simulink model "Catch_traffic_light_ver05_sushi_201222"  (R2019b)
settings: Solver=ode1  StartTime=0.0  StopTime=inf  FixedStep=0.001  RelTol=1e-3
PreLoadFcn:
  | vehicle = 'Car'; if ~length(which('cmself')), cmenv; end
  | Catch_traffic_light_ver02_sushi_201217_bus
InitFcn:
  | vehicle = 'Car'; if ~length(which('cmself')), cmenv; end
  | Catch_traffic_light_ver02_sushi_201217_bus
libraries: CarMaker4SL x45, simulink x3
Description:
  | CarMaker Plug-in Model Target
settings Model: Creator=ambl  LastModifiedBy=ambl
settings RTWCC: Description=CarMaker Plug-in Model Target  SystemTargetFile=CarMaker.tlc  TemplateMakefile=CarMaker_unix-linux64.tmf
settings CodeAppCC: MaxIdLength=127
settings STFCustomTargetCC: TargetLangStandard=C99 (ISO)  CombineOutputUpdateFcns=on  MultiInstanceERTCode=on  CodeInterfacePackaging=Reusable function  GenerateAllocFcn=on  SystemTargetFile=CarMaker.tlc
settings GRTTargetCC: ParMdlRefBuildCompliant=off  CompOptLevelCompliant=off  ConcurrentExecutionCompliant=off  MatFileLogging=off  MultiInstanceERTCode=on  CodeInterfacePackaging=Reusable function  CPPClassGenCompliant=off  GenerateAllocFcn=on  UseToolchainInfoCompliant=off

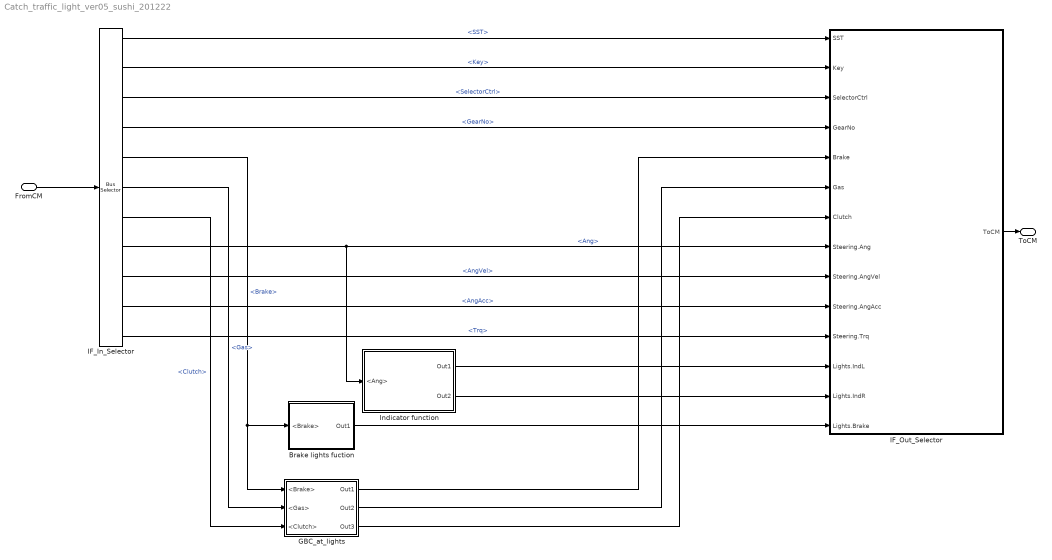
== system Catch_traffic_light_ver05_sushi_201222 ==
  FromCM : Inport  OutDataTypeStr=Bus: cmVehicleControlIn
  Brake lights fuction : Subsystem
  GBC_at_lights : Subsystem
  IF_In_Selector : BusSelector  OutputSignals=SST,Key,SelectorCtrl,GearNo,Brake,Gas,Clutch,Steering.Ang,Steering.AngVel,Steering.AngAcc,Steering.Trq
  IF_Out_Selector : Subsystem  mask(Signal Selection){}
      mask help: Signal Selection Block
      settings: OpenFcn=cmSignalSelect('SignalSelection_CB',gcb)
  Indicator function : Subsystem
  ToCM : Outport  OutDataTypeStr=Bus: cmVehicleControlOut
  wires:
  FromCM/1 -> IF_In_Selector/1
  IF_Out_Selector/1(ToCM) -> ToCM/1
  IF_In_Selector/1 -> IF_Out_Selector/1(SST)  "<SST>"
  IF_In_Selector/2 -> IF_Out_Selector/2(Key)  "<Key>"
  IF_In_Selector/3 -> IF_Out_Selector/3(SelectorCtrl)  "<SelectorCtrl>"
  IF_In_Selector/5 -> Brake lights fuction/1(<Brake>), GBC_at_lights/1(<Brake>)  "<Brake>"
  IF_In_Selector/8 -> IF_Out_Selector/8(Steering.Ang), Indicator function/1("<Ang> ")  "<Ang>"
  IF_In_Selector/9 -> IF_Out_Selector/9(Steering.AngVel)  "<AngVel>"
  IF_In_Selector/10 -> IF_Out_Selector/10(Steering.AngAcc)  "<AngAcc>"
  IF_In_Selector/11 -> IF_Out_Selector/11(Steering.Trq)  "<Trq>"
  Brake lights fuction/1(Out1) -> IF_Out_Selector/14(Lights.Brake)
  Indicator function/1(Out1) -> IF_Out_Selector/12(Lights.IndL)
  Indicator function/2(Out2) -> IF_Out_Selector/13(Lights.IndR)
  IF_In_Selector/6 -> GBC_at_lights/2(<Gas>)  "<Gas>"
  IF_In_Selector/7 -> GBC_at_lights/3(<Clutch>)  "<Clutch>"
  GBC_at_lights/3(Out3) -> IF_Out_Selector/7(Clutch)
  GBC_at_lights/2(Out2) -> IF_Out_Selector/6(Gas)
  GBC_at_lights/1(Out1) -> IF_Out_Selector/5(Brake)
  IF_In_Selector/4 -> IF_Out_Selector/4(GearNo)  "<GearNo>"

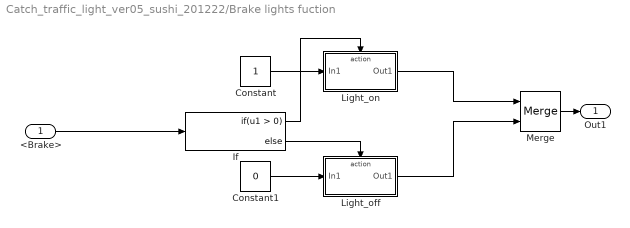
== system Catch_traffic_light_ver05_sushi_201222/Brake lights fuction ==
  <Brake> : Inport
  Constant : Constant
  Constant1 : Constant  Value=0
  If : If
  Light_off : Subsystem  TreatAsAtomicUnit=on
  Light_on : Subsystem  TreatAsAtomicUnit=on
  Merge : Merge
  Out1 : Outport
  wires:
  If/2 -> Light_off/Action
  Constant1/1 -> Light_off/1(In1)
  Merge/1 -> Out1/1
  Constant/1 -> Light_on/1(In1)
  <Brake>/1 -> If/1
  Light_on/1(Out1) -> Merge/1
  Light_off/1(Out1) -> Merge/2
  If/1 -> Light_on/Action

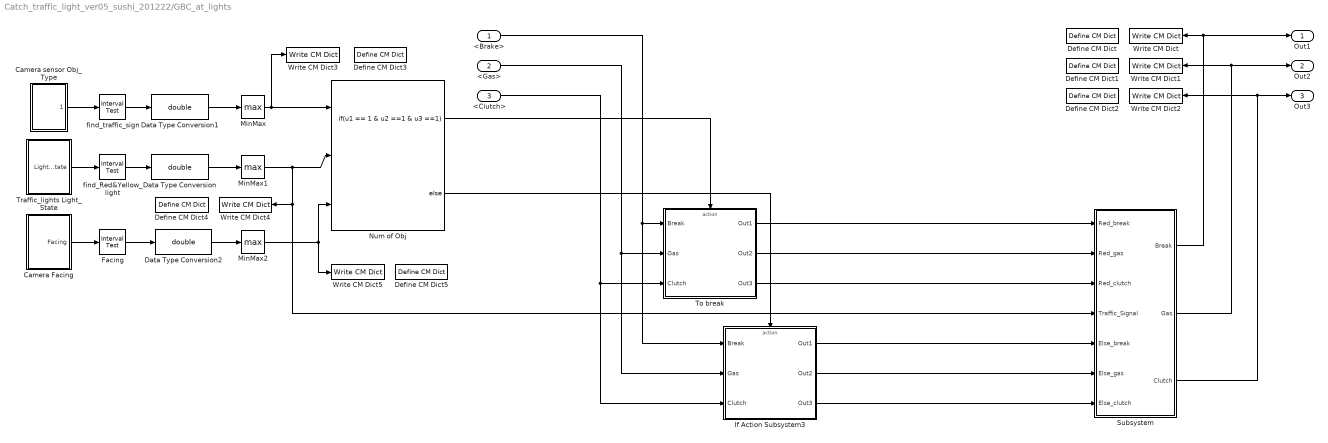
== system Catch_traffic_light_ver05_sushi_201222/GBC_at_lights ==
  <Brake> : Inport
  <Gas> : Inport  Port=2
  <Clutch> : Inport  Port=3
  Camera Facing : Subsystem
  Camera sensor Obj_Type : Subsystem
  Data Type Conversion : DataTypeConversion  OutDataTypeStr=double
  Data Type Conversion1 : DataTypeConversion  OutDataTypeStr=double
  Data Type Conversion2 : DataTypeConversion  OutDataTypeStr=double
  Define CM Dict : CarMaker4SL/Define CM Dict  xname=ctrl_break  xmono=off  xtype=Double4  xdvaplace=None  xnstates=0  xfirststate=0  xinitial=0
  Define CM Dict1 : CarMaker4SL/Define CM Dict  xname=ctrl_gas  xmono=off  xtype=Double4  xdvaplace=None  xnstates=0  xfirststate=0  xinitial=0
  Define CM Dict2 : CarMaker4SL/Define CM Dict  xname=ctrl_clutch  xmono=off  xtype=Double4  xdvaplace=None  xnstates=0  xfirststate=0  xinitial=0
  Define CM Dict3 : CarMaker4SL/Define CM Dict  xname=ctrl_obj_type  xmono=off  xtype=Double4  xdvaplace=None  xnstates=0  xfirststate=0  xinitial=0
  Define CM Dict4 : CarMaker4SL/Define CM Dict  xname=ctrl_light_state  xmono=off  xtype=Double4  xdvaplace=None  xnstates=0  xfirststate=0  xinitial=0
  Define CM Dict5 : CarMaker4SL/Define CM Dict  xname=ctrl_facing  xmono=off  xtype=Double4  xdvaplace=None  xnstates=0  xfirststate=0  xinitial=0
  Facing : simulink/Logic and Bit Operations/Interval Test  IntervalClosedRight=on  uplimit=1.5  IntervalClosedLeft=on  lowlimit=0.5  OutDataTypeStr=boolean
  If Action Subsystem3 : Subsystem  TreatAsAtomicUnit=on
  MinMax : MinMax  Function=max
  MinMax1 : MinMax  Function=max
  MinMax2 : MinMax  Function=max
  Num of Obj : If  NumInputs=3  IfExpression=u1 == 1 & u2 ==1 & u3 ==1
  Subsystem : Subsystem
  To break : Subsystem  TreatAsAtomicUnit=on
  Traffic_lights Light_State : Subsystem
  Write CM Dict : CarMaker4SL/Write CM Dict  xname=ctrl_break  xsync=off
  Write CM Dict1 : CarMaker4SL/Write CM Dict  xname=ctrl_gas  xsync=off
  Write CM Dict2 : CarMaker4SL/Write CM Dict  xname=ctrl_clutch  xsync=off
  Write CM Dict3 : CarMaker4SL/Write CM Dict  xname=ctrl_obj_type  xsync=off
  Write CM Dict4 : CarMaker4SL/Write CM Dict  xname=ctrl_light_state  xsync=off
  Write CM Dict5 : CarMaker4SL/Write CM Dict  xname=ctrl_facing  xsync=off
  find_Red&Yellow_light : simulink/Logic and Bit Operations/Interval Test  IntervalClosedRight=on  uplimit=3.5  IntervalClosedLeft=on  lowlimit=2.5  OutDataTypeStr=boolean
  find_traffic_sign : simulink/Logic and Bit Operations/Interval Test  IntervalClosedRight=on  uplimit=5.5  IntervalClosedLeft=on  lowlimit=4.5  OutDataTypeStr=boolean
  Out1 : Outport
  Out2 : Outport  Port=2
  Out3 : Outport  Port=3
  wires:
  Subsystem/2(Gas) -> Write CM Dict1/1, Out2/1
  Subsystem/1(Break) -> Write CM Dict/1, Out1/1
  Subsystem/3(Clutch) -> Write CM Dict2/1, Out3/1
  If Action Subsystem3/1(Out1) -> Subsystem/5(Else_break)
  If Action Subsystem3/2(Out2) -> Subsystem/6("Else_gas ")
  If Action Subsystem3/3(Out3) -> Subsystem/7("Else_clutch ")
  To break/1(Out1) -> Subsystem/1(Red_break)
  To break/2(Out2) -> Subsystem/2(Red_gas)
  To break/3(Out3) -> Subsystem/3(Red_clutch)
  Num of Obj/1 -> To break/Action
  Num of Obj/2 -> If Action Subsystem3/Action
  <Gas>/1 -> If Action Subsystem3/2(Gas), To break/2(Gas)
  <Brake>/1 -> If Action Subsystem3/1(Break), To break/1(Break)
  <Clutch>/1 -> If Action Subsystem3/3(Clutch), To break/3(Clutch)
  find_traffic_sign/1 -> Data Type Conversion1/1
  Camera sensor Obj_Type/1(Obj_Type) -> find_traffic_sign/1
  Traffic_lights Light_State/1(Light_State) -> find_Red&Yellow_light/1
  MinMax/1 -> Write CM Dict3/1, Num of Obj/1
  MinMax1/1 -> Subsystem/4(Traffic_Signal), Write CM Dict4/1, Num of Obj/2
  Data Type Conversion1/1 -> MinMax/1
  find_Red&Yellow_light/1 -> Data Type Conversion/1
  Data Type Conversion/1 -> MinMax1/1
  Camera Facing/1(Facing) -> Facing/1
  Facing/1 -> Data Type Conversion2/1
  Data Type Conversion2/1 -> MinMax2/1
  MinMax2/1 -> Write CM Dict5/1, Num of Obj/3

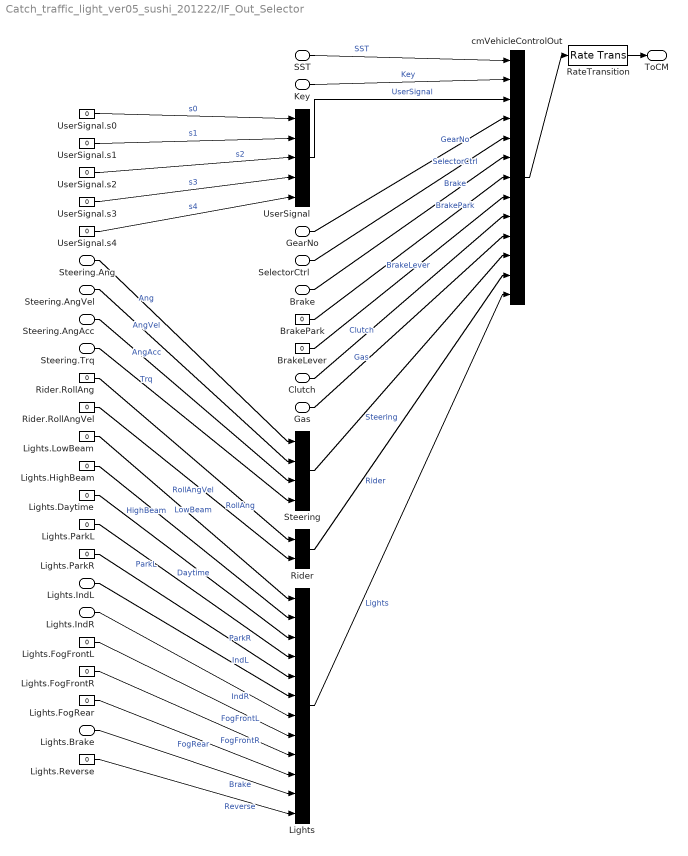
== system Catch_traffic_light_ver05_sushi_201222/IF_Out_Selector ==
  SST : Inport
  Key : Inport  Port=2
  SelectorCtrl : Inport  Port=3
  GearNo : Inport  Port=4
  Brake : Inport  Port=5
  Gas : Inport  Port=6
  Clutch : Inport  Port=7
  Steering.Ang : Inport  Port=8
  Steering.AngVel : Inport  Port=9
  Steering.AngAcc : Inport  Port=10
  Steering.Trq : Inport  Port=11
  Lights.IndL : Inport  Port=12
  Lights.IndR : Inport  Port=13
  Lights.Brake : Inport  Port=14
  BrakeLever : Constant  Value=0
  BrakePark : Constant  Value=0
  Lights : BusCreator  Inputs=12
  Lights.Daytime : Constant  Value=0
  Lights.FogFrontL : Constant  Value=0
  Lights.FogFrontR : Constant  Value=0
  Lights.FogRear : Constant  Value=0
  Lights.HighBeam : Constant  Value=0
  Lights.LowBeam : Constant  Value=0
  Lights.ParkL : Constant  Value=0
  Lights.ParkR : Constant  Value=0
  Lights.Reverse : Constant  Value=0
  RateTransition : RateTransition  OutPortSampleTime=str2num(get_param(bdroot,'FixedStep'))
  Rider : BusCreator  Inputs=2
  Rider.RollAng : Constant  Value=0
  Rider.RollAngVel : Constant  Value=0
  Steering : BusCreator  Inputs=4
  UserSignal : BusCreator  Inputs=5
  UserSignal.s{0..4} (5 alike) : Constant  Value=0
  cmVehicleControlOut : BusCreator  Inputs=13
  ToCM : Outport
  wires:
  RateTransition/1 -> ToCM/1
  cmVehicleControlOut/1 -> RateTransition/1
  UserSignal/1 -> cmVehicleControlOut/3  "UserSignal"
  UserSignal.s0/1 -> UserSignal/1  "s0"
  UserSignal.s1/1 -> UserSignal/2  "s1"
  UserSignal.s2/1 -> UserSignal/3  "s2"
  UserSignal.s3/1 -> UserSignal/4  "s3"
  UserSignal.s4/1 -> UserSignal/5  "s4"
  BrakePark/1 -> cmVehicleControlOut/7  "BrakePark"
  BrakeLever/1 -> cmVehicleControlOut/8  "BrakeLever"
  Steering/1 -> cmVehicleControlOut/11  "Steering"
  Rider/1 -> cmVehicleControlOut/12  "Rider"
  Rider.RollAng/1 -> Rider/1  "RollAng"
  Rider.RollAngVel/1 -> Rider/2  "RollAngVel"
  Lights/1 -> cmVehicleControlOut/13  "Lights"
  Lights.LowBeam/1 -> Lights/1  "LowBeam"
  Lights.HighBeam/1 -> Lights/2  "HighBeam"
  Lights.Daytime/1 -> Lights/3  "Daytime"
  Lights.ParkL/1 -> Lights/4  "ParkL"
  Lights.ParkR/1 -> Lights/5  "ParkR"
  Lights.FogFrontL/1 -> Lights/8  "FogFrontL"
  Lights.FogFrontR/1 -> Lights/9  "FogFrontR"
  Lights.FogRear/1 -> Lights/10  "FogRear"
  Lights.Reverse/1 -> Lights/12  "Reverse"
  SST/1 -> cmVehicleControlOut/1  "SST"
  Key/1 -> cmVehicleControlOut/2  "Key"
  GearNo/1 -> cmVehicleControlOut/4  "GearNo"
  SelectorCtrl/1 -> cmVehicleControlOut/5  "SelectorCtrl"
  Brake/1 -> cmVehicleControlOut/6  "Brake"
  Clutch/1 -> cmVehicleControlOut/9  "Clutch"
  Gas/1 -> cmVehicleControlOut/10  "Gas"
  Steering.Ang/1 -> Steering/1  "Ang"
  Steering.AngVel/1 -> Steering/2  "AngVel"
  Steering.AngAcc/1 -> Steering/3  "AngAcc"
  Steering.Trq/1 -> Steering/4  "Trq"
  Lights.IndL/1 -> Lights/6  "IndL"
  Lights.IndR/1 -> Lights/7  "IndR"
  Lights.Brake/1 -> Lights/11  "Brake"

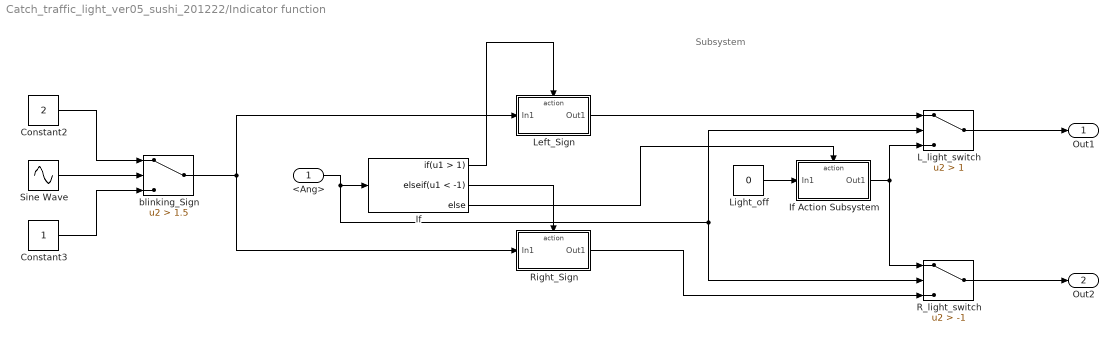
== system Catch_traffic_light_ver05_sushi_201222/Indicator function ==
  note: Subsystem
  "<Ang> " : Inport
  Constant2 : Constant  Value=2
  Constant3 : Constant
  If : If  IfExpression=u1 > 1  ElseIfExpressions=u1 < -1
  If Action Subsystem : Subsystem  TreatAsAtomicUnit=on
  L_light_switch : Switch  Criteria=u2 > Threshold  Threshold=1
  Left_Sign : Subsystem  TreatAsAtomicUnit=on
  Light_off : Constant  Value=0
  R_light_switch : Switch  Criteria=u2 > Threshold  Threshold=-1
  Right_Sign : Subsystem  TreatAsAtomicUnit=on
  Sine Wave : Sin  Amplitude=0.5  Bias=1.5  Frequency=4.71  SampleTime=0
  blinking_Sign : Switch  Criteria=u2 > Threshold  Threshold=1.5
  Out1 : Outport
  Out2 : Outport  Port=2
  wires:
  If/1 -> Left_Sign/Action
  Sine Wave/1 -> blinking_Sign/2
  Constant2/1 -> blinking_Sign/1
  Constant3/1 -> blinking_Sign/3
  blinking_Sign/1 -> Left_Sign/1(In1), Right_Sign/1(In1)
  If/2 -> Right_Sign/Action
  L_light_switch/1 -> Out1/1
  R_light_switch/1 -> Out2/1
  "<Ang> "/1 -> L_light_switch/2, R_light_switch/2, If/1
  Light_off/1 -> If Action Subsystem/1(In1)
  If Action Subsystem/1(Out1) -> R_light_switch/1, L_light_switch/3
  Right_Sign/1(Out1) -> R_light_switch/3
  Left_Sign/1(Out1) -> L_light_switch/1
  If/3 -> If Action Subsystem/Action

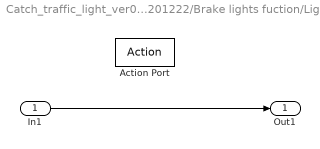
== system Catch_traffic_light_ver05_sushi_201222/Brake lights fuction/Light_off ==
  In1 : Inport
  Action Port : ActionPort  ActionPortLabel=else
  Out1 : Outport
  wires:
  In1/1 -> Out1/1

== system Catch_traffic_light_ver05_sushi_201222/Brake lights fuction/Light_on ==
  In1 : Inport
  Action Port : ActionPort  ActionPortLabel=if(u1 > 0)
  Out1 : Outport
  wires:
  In1/1 -> Out1/1

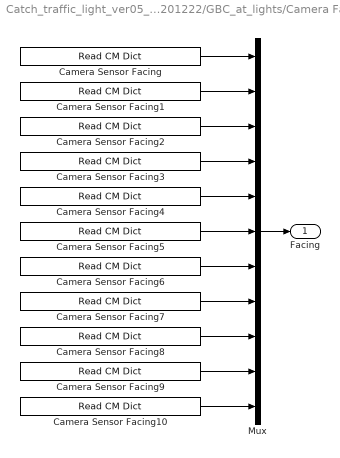
== system Catch_traffic_light_ver05_sushi_201222/GBC_at_lights/Camera Facing ==
  Camera Sensor Facing : CarMaker4SL/Read CM Dict  xname=Sensor.Camera.CA00.Obj.0.Facing  xsync=off
  Camera Sensor Facing1 : CarMaker4SL/Read CM Dict  xname=Sensor.Camera.CA00.Obj.1.Facing  xsync=off
  Camera Sensor Facing10 : CarMaker4SL/Read CM Dict  xname=Sensor.Camera.CA00.Obj.10.Facing  xsync=off
  Camera Sensor Facing2 : CarMaker4SL/Read CM Dict  xname=Sensor.Camera.CA00.Obj.2.Facing  xsync=off
  Camera Sensor Facing3 : CarMaker4SL/Read CM Dict  xname=Sensor.Camera.CA00.Obj.3.Facing  xsync=off
  Camera Sensor Facing4 : CarMaker4SL/Read CM Dict  xname=Sensor.Camera.CA00.Obj.4.Facing  xsync=off
  Camera Sensor Facing5 : CarMaker4SL/Read CM Dict  xname=Sensor.Camera.CA00.Obj.5.Facing  xsync=off
  Camera Sensor Facing6 : CarMaker4SL/Read CM Dict  xname=Sensor.Camera.CA00.Obj.6.Facing  xsync=off
  Camera Sensor Facing7 : CarMaker4SL/Read CM Dict  xname=Sensor.Camera.CA00.Obj.7.Facing  xsync=off
  Camera Sensor Facing8 : CarMaker4SL/Read CM Dict  xname=Sensor.Camera.CA00.Obj.8.Facing  xsync=off
  Camera Sensor Facing9 : CarMaker4SL/Read CM Dict  xname=Sensor.Camera.CA00.Obj.9.Facing  xsync=off
  Mux : Mux  Inputs=11
  Facing : Outport
  wires:
  Camera Sensor Facing/1 -> Mux/1
  Camera Sensor Facing1/1 -> Mux/2
  Camera Sensor Facing2/1 -> Mux/3
  Camera Sensor Facing3/1 -> Mux/4
  Camera Sensor Facing4/1 -> Mux/5
  Camera Sensor Facing5/1 -> Mux/6
  Camera Sensor Facing6/1 -> Mux/7
  Camera Sensor Facing7/1 -> Mux/8
  Camera Sensor Facing8/1 -> Mux/9
  Camera Sensor Facing9/1 -> Mux/10
  Camera Sensor Facing10/1 -> Mux/11
  Mux/1 -> Facing/1

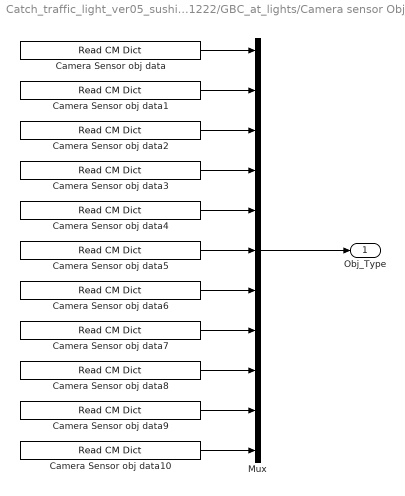
== system Catch_traffic_light_ver05_sushi_201222/GBC_at_lights/Camera sensor Obj_Type ==
  Camera Sensor obj data : CarMaker4SL/Read CM Dict  xname=Sensor.Camera.CA00.Obj.0.Type  xsync=off
  Camera Sensor obj data1 : CarMaker4SL/Read CM Dict  xname=Sensor.Camera.CA00.Obj.1.Type  xsync=off
  Camera Sensor obj data10 : CarMaker4SL/Read CM Dict  xname=Sensor.Camera.CA00.Obj.10.Type  xsync=off
  Camera Sensor obj data2 : CarMaker4SL/Read CM Dict  xname=Sensor.Camera.CA00.Obj.2.Type  xsync=off
  Camera Sensor obj data3 : CarMaker4SL/Read CM Dict  xname=Sensor.Camera.CA00.Obj.3.Type  xsync=off
  Camera Sensor obj data4 : CarMaker4SL/Read CM Dict  xname=Sensor.Camera.CA00.Obj.4.Type  xsync=off
  Camera Sensor obj data5 : CarMaker4SL/Read CM Dict  xname=Sensor.Camera.CA00.Obj.5.Type  xsync=off
  Camera Sensor obj data6 : CarMaker4SL/Read CM Dict  xname=Sensor.Camera.CA00.Obj.6.Type  xsync=off
  Camera Sensor obj data7 : CarMaker4SL/Read CM Dict  xname=Sensor.Camera.CA00.Obj.7.Type  xsync=off
  Camera Sensor obj data8 : CarMaker4SL/Read CM Dict  xname=Sensor.Camera.CA00.Obj.8.Type  xsync=off
  Camera Sensor obj data9 : CarMaker4SL/Read CM Dict  xname=Sensor.Camera.CA00.Obj.9.Type  xsync=off
  Mux : Mux  Inputs=11
  Obj_Type : Outport
  wires:
  Camera Sensor obj data6/1 -> Mux/7
  Camera Sensor obj data7/1 -> Mux/8
  Camera Sensor obj data3/1 -> Mux/4
  Camera Sensor obj data/1 -> Mux/1
  Camera Sensor obj data5/1 -> Mux/6
  Camera Sensor obj data2/1 -> Mux/3
  Camera Sensor obj data10/1 -> Mux/11
  Camera Sensor obj data1/1 -> Mux/2
  Camera Sensor obj data8/1 -> Mux/9
  Camera Sensor obj data4/1 -> Mux/5
  Camera Sensor obj data9/1 -> Mux/10
  Mux/1 -> Obj_Type/1

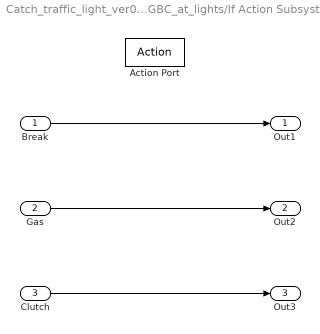
== system Catch_traffic_light_ver05_sushi_201222/GBC_at_lights/If Action Subsystem3 ==
  Break : Inport
  Gas : Inport  Port=2
  Clutch : Inport  Port=3
  Action Port : ActionPort  ActionPortLabel=else
  Out1 : Outport
  Out2 : Outport  Port=2
  Out3 : Outport  Port=3
  wires:
  Break/1 -> Out1/1
  Gas/1 -> Out2/1
  Clutch/1 -> Out3/1

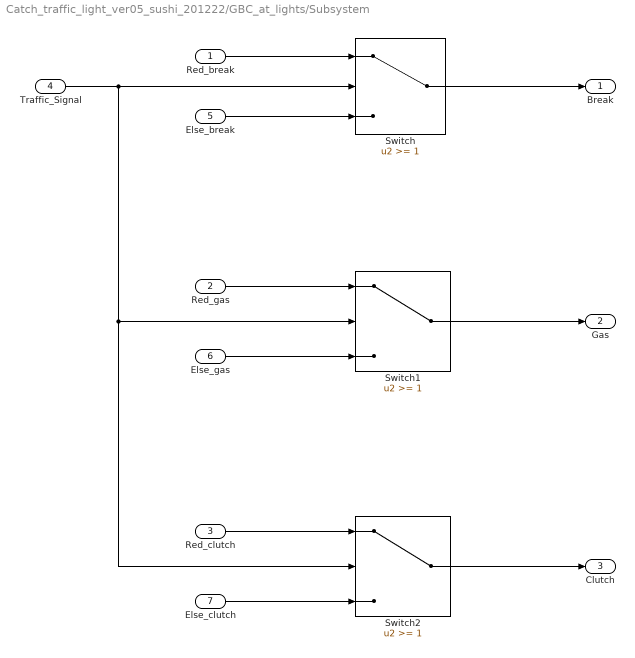
== system Catch_traffic_light_ver05_sushi_201222/GBC_at_lights/Subsystem ==
  Red_break : Inport
  Red_gas : Inport  Port=2
  Red_clutch : Inport  Port=3
  Traffic_Signal : Inport  Port=4
  Else_break : Inport  Port=5
  "Else_gas " : Inport  Port=6
  "Else_clutch " : Inport  Port=7
  Switch : Switch  Threshold=1
  Switch1 : Switch  Threshold=1
  Switch2 : Switch  Threshold=1
  Break : Outport
  Gas : Outport  Port=2
  Clutch : Outport  Port=3
  wires:
  Traffic_Signal/1 -> Switch2/2, Switch1/2, Switch/2
  Else_break/1 -> Switch/3
  Red_break/1 -> Switch/1
  Switch/1 -> Break/1
  Red_gas/1 -> Switch1/1
  "Else_gas "/1 -> Switch1/3
  Switch1/1 -> Gas/1
  Red_clutch/1 -> Switch2/1
  "Else_clutch "/1 -> Switch2/3
  Switch2/1 -> Clutch/1

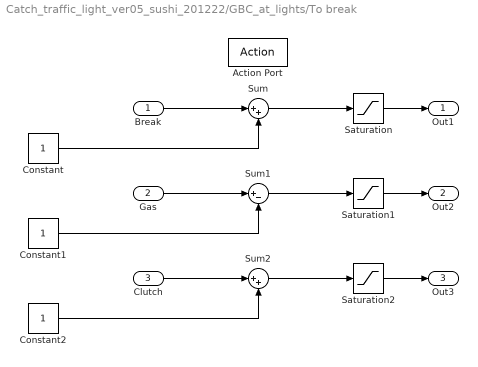
== system Catch_traffic_light_ver05_sushi_201222/GBC_at_lights/To break ==
  Break : Inport
  Gas : Inport  Port=2
  Clutch : Inport  Port=3
  Action Port : ActionPort  ActionPortLabel=if(u1 == 1 & u2 ==1 & u3 ==1)
  Constant : Constant
  Constant1 : Constant
  Constant2 : Constant
  Saturation : Saturate  UpperLimit=1  LowerLimit=0
  Saturation1 : Saturate  UpperLimit=1  LowerLimit=0
  Saturation2 : Saturate  UpperLimit=1  LowerLimit=0
  Sum : Sum  Inputs=|++
  Sum1 : Sum  Inputs=|+-
  Sum2 : Sum  Inputs=|++
  Out1 : Outport
  Out2 : Outport  Port=2
  Out3 : Outport  Port=3
  wires:
  Saturation/1 -> Out1/1
  Saturation1/1 -> Out2/1
  Saturation2/1 -> Out3/1
  Constant/1 -> Sum/2
  Sum/1 -> Saturation/1
  Break/1 -> Sum/1
  Gas/1 -> Sum1/1
  Sum1/1 -> Saturation1/1
  Constant1/1 -> Sum1/2
  Clutch/1 -> Sum2/1
  Sum2/1 -> Saturation2/1
  Constant2/1 -> Sum2/2

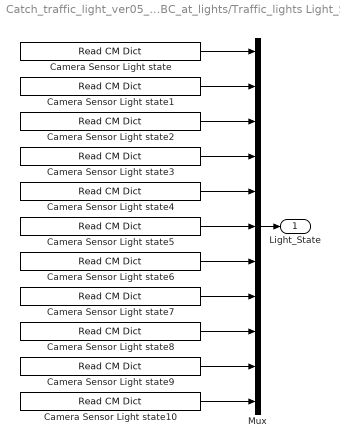
== system Catch_traffic_light_ver05_sushi_201222/GBC_at_lights/Traffic_lights Light_State ==
  Camera Sensor Light state : CarMaker4SL/Read CM Dict  xname=Sensor.Camera.CA00.Obj.0.LightState  xsync=off
  Camera Sensor Light state1 : CarMaker4SL/Read CM Dict  xname=Sensor.Camera.CA00.Obj.1.LightState  xsync=off
  Camera Sensor Light state10 : CarMaker4SL/Read CM Dict  xname=Sensor.Camera.CA00.Obj.10.LightState  xsync=off
  Camera Sensor Light state2 : CarMaker4SL/Read CM Dict  xname=Sensor.Camera.CA00.Obj.2.LightState  xsync=off
  Camera Sensor Light state3 : CarMaker4SL/Read CM Dict  xname=Sensor.Camera.CA00.Obj.3.LightState  xsync=off
  Camera Sensor Light state4 : CarMaker4SL/Read CM Dict  xname=Sensor.Camera.CA00.Obj.4.LightState  xsync=off
  Camera Sensor Light state5 : CarMaker4SL/Read CM Dict  xname=Sensor.Camera.CA00.Obj.5.LightState  xsync=off
  Camera Sensor Light state6 : CarMaker4SL/Read CM Dict  xname=Sensor.Camera.CA00.Obj.6.LightState  xsync=off
  Camera Sensor Light state7 : CarMaker4SL/Read CM Dict  xname=Sensor.Camera.CA00.Obj.7.LightState  xsync=off
  Camera Sensor Light state8 : CarMaker4SL/Read CM Dict  xname=Sensor.Camera.CA00.Obj.8.LightState  xsync=off
  Camera Sensor Light state9 : CarMaker4SL/Read CM Dict  xname=Sensor.Camera.CA00.Obj.9.LightState  xsync=off
  Mux : Mux  Inputs=11
  Light_State : Outport
  wires:
  Camera Sensor Light state9/1 -> Mux/10
  Mux/1 -> Light_State/1
  Camera Sensor Light state/1 -> Mux/1
  Camera Sensor Light state7/1 -> Mux/8
  Camera Sensor Light state1/1 -> Mux/2
  Camera Sensor Light state4/1 -> Mux/5
  Camera Sensor Light state2/1 -> Mux/3
  Camera Sensor Light state6/1 -> Mux/7
  Camera Sensor Light state8/1 -> Mux/9
  Camera Sensor Light state10/1 -> Mux/11
  Camera Sensor Light state5/1 -> Mux/6
  Camera Sensor Light state3/1 -> Mux/4

== system Catch_traffic_light_ver05_sushi_201222/Indicator function/If Action Subsystem ==
  In1 : Inport
  Action Port : ActionPort  ActionPortLabel=else
  Out1 : Outport
  wires:
  In1/1 -> Out1/1

== system Catch_traffic_light_ver05_sushi_201222/Indicator function/Left_Sign ==
  In1 : Inport
  Action Port : ActionPort  ActionPortLabel=if(u1 > 1)
  Out1 : Outport
  wires:
  In1/1 -> Out1/1

== system Catch_traffic_light_ver05_sushi_201222/Indicator function/Right_Sign ==
  In1 : Inport
  Action Port : ActionPort  ActionPortLabel=elseif(u1 < -1)
  Out1 : Outport
  wires:
  In1/1 -> Out1/1
